simulink model "LDPC"  (R2019b)
settings: Solver=VariableStepAuto  StartTime=0.0  StopTime=10.0  RelTol=1e-3
undefined symbols (not defined in the file or in its folder): dvbs2ldpc, EbNo
libraries: commsink2 x2, commblkcod2 x2, commdigbbndpm3 x2, commchan3 x1, commrandsrc3 x1
settings Model: Creator=jose_  LastModifiedBy=jose_

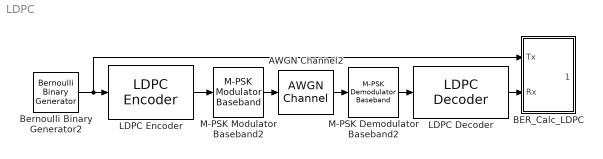
== system LDPC ==
  AWGN Channel2 : commchan3/AWGN Channel  InputProcessing=Columns as channels (frame based)  seed=67  noiseMode="Signal to noise ratio  (Eb/No)"  EbNodB=EbNo  EsNodB=10  SNRdB=EbNo  bitsPerSym=2  Ps=1  Tsym=0.01  variance=1
      settings: SourceProductName=Communications Toolbox
  BER_Calc_LDPC : Subsystem
  Bernoulli Binary Generator2 : commrandsrc3/Bernoulli Binary Generator  ProbabilityOfZero=0.5  SeedSource=Auto  Seed=0  SampleTime=0.01  SamplesPerFrame=32400  OutputDataType=double  SimulateUsing=Interpreted execution
      settings: SourceProductName=Communications Toolbox
  LDPC Decoder : commblkcod2/LDPC Decoder  ParityCheckMat=dvbs2ldpc(1/2)  OutputFmt=Information part  DecisionType=Hard decision  OutputDataType=double  NumIter=50  DoParityCheck=on  OutputNumIter=off  OutputFinalChecks=off
      settings: SourceProductName=Communications Toolbox  SourceProductBaseCode=CM
  LDPC Encoder : commblkcod2/LDPC Encoder  ParityCheckMat=dvbs2ldpc(1/2)
      settings: SourceProductName=Communications Toolbox  SourceProductBaseCode=CM
  M-PSK Demodulator Baseband2 : commdigbbndpm3/M-PSK Demodulator Baseband  M=4  OutType=Bit  DecType=Approximate log-likelihood ratio  VarSource=Dialog  Variance=db2pow(EbNo)  Dec=Gray  Mapping=[0:7]  Ph=0  outDtype1=Inherit via internal rule  outDtype2=Inherit via internal rule  derotateFactorWordLen=16  derotateFactorDataTypeStr=Inherit: Same word length as input  derotateFactorLastDataTypeStr=Inherit: Same word length as input
      settings: SourceProductName=Communications Toolbox
  M-PSK Modulator Baseband2 : commdigbbndpm3/M-PSK Modulator Baseband  M=4  InType=Bit  Enc=Gray  Mapping=[0:7]  Ph=0  outDtype=double  outWordLen=16  outUDDataType=sfix(16)  outFracLenMode=Best precision  outFracLen=15  outDataTypeStr=double  outLastDataTypeStr=double
      settings: SourceProductName=Communications Toolbox
  wires:
  Bernoulli Binary Generator2/1 -> BER_Calc_LDPC/1(Tx), LDPC Encoder/1
  LDPC Decoder/1 -> BER_Calc_LDPC/2(Rx)
  AWGN Channel2/1 -> M-PSK Demodulator Baseband2/1
  LDPC Encoder/1 -> M-PSK Modulator Baseband2/1
  M-PSK Demodulator Baseband2/1 -> LDPC Decoder/1
  M-PSK Modulator Baseband2/1 -> AWGN Channel2/1

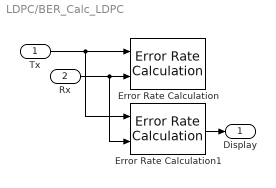
== system LDPC/BER_Calc_LDPC ==
  Tx : Inport
  Rx : Inport  Port=2
  Error Rate Calculation : commsink2/Error Rate Calculation  N=0  st_delay=0  cp_mode=Entire frame  subframe=[]  PMode=Workspace  WsName=LDPCError  RsMode2=off  stop=off  numErr=100  maxBits=1e6
      settings: SourceProductName=Communications Toolbox
  Error Rate Calculation1 : commsink2/Error Rate Calculation  N=0  st_delay=0  cp_mode=Entire frame  subframe=[]  PMode=Port  WsName=ErrorVec  RsMode2=off  stop=off  numErr=100  maxBits=1e6
      settings: SourceProductName=Communications Toolbox
  Display : Outport
  wires:
  Rx/1 -> Error Rate Calculation1/2, Error Rate Calculation/2
  Tx/1 -> Error Rate Calculation1/1, Error Rate Calculation/1
  Error Rate Calculation1/1 -> Display/1
